simulink model "dragFallBall"  (R2022b)
settings: Solver=ode45  StartTime=0.0  StopTime=10.0  RelTol=1e-3  EnableMultiTasking=on
PreLoadFcn:
  | ballParams
values from neighbouring files (symbols this model uses):
  A = pi*d^2/4    (= 0.00441786466911)    [ballParams.m]    (also in bungeeParams.m = 0.5)
  CD = 0.3    [ballParams.m]    (also in bmwParams.m = 0.4; bungeeParams.m = 0.6)
  m = 0.145    [ballParams.m]    (also in bmwParams.m = 104.2; bungeeParams.m = 90)
  rho = 1.2    [ballParams.m]    (also in bmwParams.m = 0.002377; bungeeParams.m)
settings Model: Creator=jrivitus  LastModifiedBy=bensweet
settings SolverCC: AlgebraicLoopSolver=TrustRegion
settings DataIOCC: LimitDataPoints=on  SaveFormat=Array  ReturnWorkspaceOutputs=off
settings OptimizationCC: ExpressionDepthLimit=2147483647  InitFltsAndDblsToZero=on  LifeSpan=inf
settings DebuggingCC: UnconnectedInputMsg=warning  UnconnectedOutputMsg=warning  UnconnectedLineMsg=warning  PregeneratedLibrarySubsystemCodeDiagnostic=none  SFMachineParentedDataDiag=warning
settings HardwareCC: ProdBitPerPointer=32  ProdBitPerSizeT=32  ProdBitPerPtrDiffT=32  ProdLargestAtomicFloat=None  ProdIntDivRoundTo=Undefined  ProdEndianess=Unspecified  ProdWordSize=32  ProdHWDeviceType=32-bit Generic
settings ModelReferenceCC: EnableRefExpFcnMdlSchedulingChecks=on  PropagateSignalLabelsOutOfModel=off
settings SFSimCC: SimUseLocalCustomCode=off
settings RTWCC: RTWUseLocalCustomCode=off  DLArmComputeVersion=19.05
settings CodeAppCC: StateflowObjectComments=on
settings GRTTargetCC: TargetLangStandard=C89/C90 (ANSI)  CombineOutputUpdateFcns=off  GRTInterface=on
settings ConfigComp: CovMetricSettings=dw  CovSaveCumulativeToWorkspaceVar=on  CovSaveSingleToWorkspaceVar=on  CovExternalEMLEnable=off  CovSFcnEnable=off

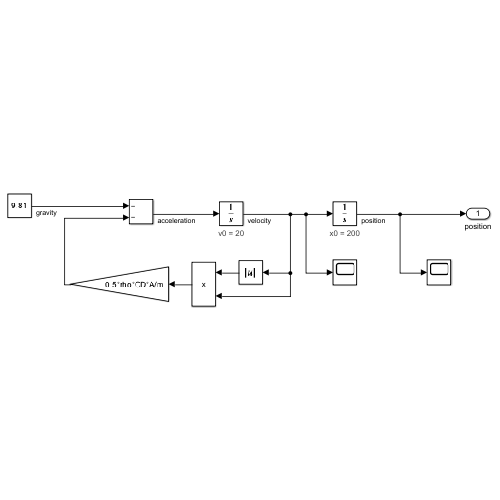
[thumbnail: Simulink's stored preview of the top-level diagram]
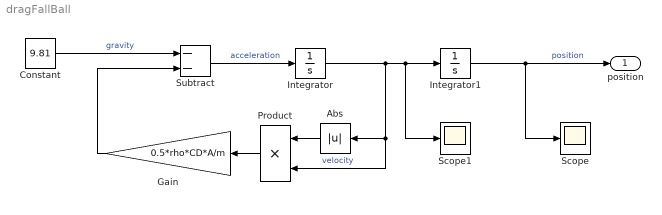
== system dragFallBall ==
  Abs : Abs  SaturateOnIntegerOverflow=off
  Constant : Constant  Value=9.81
  Gain : Gain  Gain=0.5*rho*CD*A/m
  Integrator : Integrator  InitialCondition=20
      settings: AttributesFormatString=v0 = %<InitialCondition>
  Integrator1 : Integrator  InitialCondition=200
      settings: AttributesFormatString=x0 = %<InitialCondition>
  Product : Product
  Scope : Scope
  Scope1 : Scope
  Subtract : Sum  Inputs=--
  position : Outport  VectorParamsAs1DForOutWhenUnconnected=off
  wires:
  Subtract/1 -> Integrator/1  "acceleration"
  Integrator/1 -> Product/2, Abs/1, Integrator1/1, Scope1/1  "velocity"
  Integrator1/1 -> position/1, Scope/1  "position"
  Constant/1 -> Subtract/1  "gravity"
  Gain/1 -> Subtract/2
  Abs/1 -> Product/1
  Product/1 -> Gain/1
